simulink model "PrimaryController"  (R2023a)
settings: Solver=VariableStepAuto  StartTime=0.0  StopTime=inf  RelTol=1e-3
model workspace (MAT data in the model file):
  MyTestVariable = Simulink.Parameter
  MyTestVariable.Value = 5
  MyTestVariable.DataType = 'auto'
  MyTestVariable.Min = 1
  MyTestVariable.Max = 10
  MyTestVariable.Complexity = 'real'
  MyTestVariable.Dimensions = [1 1]
libraries: arduinolib x20, simulink x2
settings Model: Creator=Josh Lendi  LastModifiedBy=alanl
settings DebuggingCC: UnconnectedInputMsg=warning  UnconnectedOutputMsg=warning  UnconnectedLineMsg=warning
settings ModelReferenceCC: EnableRefExpFcnMdlSchedulingChecks=on
settings RTWCC: DLArmComputeVersion=19.05

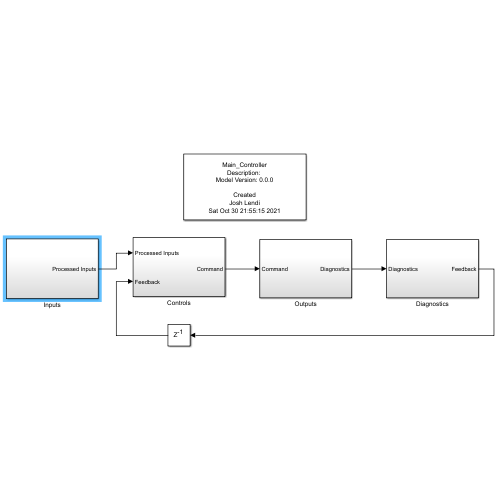
[thumbnail: Simulink's stored preview of the top-level diagram]
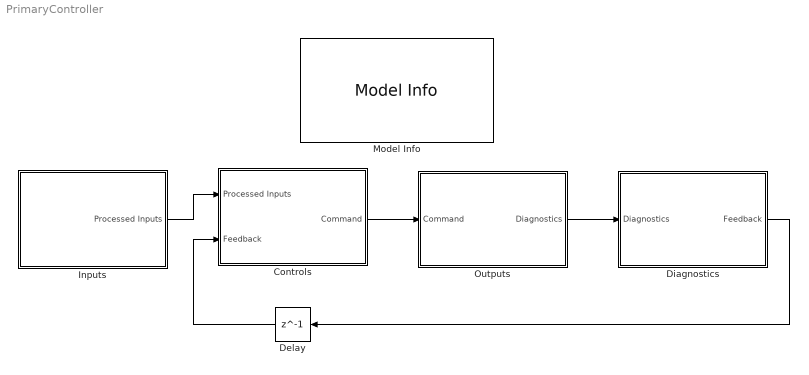
== system PrimaryController ==
  Controls : Subsystem
  Delay : Delay  DelayLength=1  InitialCondition=0
  Diagnostics : Subsystem
  Inputs : Subsystem
  Model Info : simulink/Model-Wide Utilities/Model Info  Frame=on  DisplayStringWithTags=|  HorizontalTextAlignment=Center  LeftAlignmentValue=0.5
      | %<ModelName>
      | Description: %<Description>
      | Model Version: %<ModelVersion>
      | 
      | Created
      | %<Creator>
      | %<Created>
  Outputs : Subsystem
  wires:
  Controls/1(Command) -> Outputs/1(Command)
  Outputs/1(Diagnostics) -> Diagnostics/1(Diagnostics)
  Inputs/1(Processed Inputs) -> Controls/1(Processed Inputs)
  Delay/1 -> Controls/2(Feedback)
  Diagnostics/1(Feedback) -> Delay/1

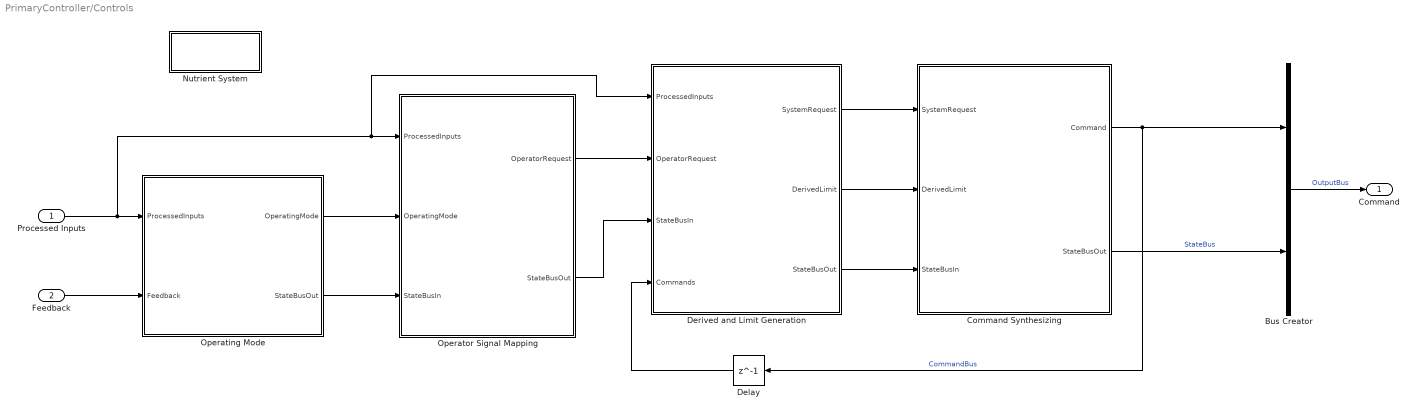
== system PrimaryController/Controls ==
  Processed Inputs : Inport
  Feedback : Inport  Port=2
  Bus Creator : BusCreator  Inputs=2
  Command Synthesizing : Subsystem
  Delay : Delay  DelayLength=1
  Derived and Limit Generation : Subsystem
  Nutrient System : Subsystem
  Operating Mode : Subsystem
  Operator Signal Mapping : Subsystem
  Command : Outport
  wires:
  Processed Inputs/1 -> Derived and Limit Generation/1(ProcessedInputs), Operator Signal Mapping/1(ProcessedInputs), Operating Mode/1(ProcessedInputs)
  Feedback/1 -> Operating Mode/2(Feedback)
  Operating Mode/1(OperatingMode) -> Operator Signal Mapping/2(OperatingMode)
  Operating Mode/2(StateBusOut) -> Operator Signal Mapping/3(StateBusIn)
  Operator Signal Mapping/1(OperatorRequest) -> Derived and Limit Generation/2(OperatorRequest)
  Operator Signal Mapping/2(StateBusOut) -> Derived and Limit Generation/3(StateBusIn)
  Derived and Limit Generation/1(SystemRequest) -> Command Synthesizing/1(SystemRequest)
  Derived and Limit Generation/2(DerivedLimit) -> Command Synthesizing/2(DerivedLimit)
  Derived and Limit Generation/3(StateBusOut) -> Command Synthesizing/3(StateBusIn)
  Command Synthesizing/2(StateBusOut) -> Bus Creator/2  "StateBus"
  Command Synthesizing/1(Command) -> Delay/1, Bus Creator/1  "CommandBus"
  Bus Creator/1 -> Command/1  "OutputBus"
  Delay/1 -> Derived and Limit Generation/4(Commands)

== system PrimaryController/Diagnostics ==
  Diagnostics : Inport
  Feedback : Outport
  wires:
  Diagnostics/1 -> Feedback/1

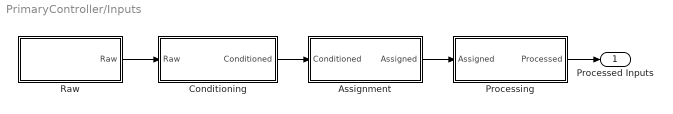
== system PrimaryController/Inputs ==
  Assignment : Subsystem
  Conditioning : Subsystem
  Processing : Subsystem
  Raw : Subsystem
  Processed Inputs : Outport
  wires:
  Raw/1(Raw) -> Conditioning/1(Raw)
  Assignment/1(Assigned) -> Processing/1(Assigned)
  Conditioning/1(Conditioned) -> Assignment/1(Conditioned)
  Processing/1(Processed) -> Processed Inputs/1

== system PrimaryController/Outputs ==
  Command : Inport
  Processing : Subsystem
  Send : Subsystem
  Diagnostics : Outport
  wires:
  Command/1 -> Processing/1(Command)
  Send/1(Diagnostic) -> Diagnostics/1
  Processing/1(Processed) -> Send/1(Processed)

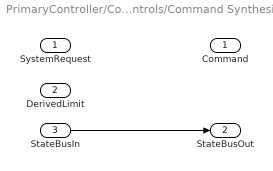
== system PrimaryController/Controls/Command Synthesizing ==
  SystemRequest : Inport
  DerivedLimit : Inport  Port=2
  StateBusIn : Inport  Port=3
  Command : Outport
  StateBusOut : Outport  Port=2
  wires:
  StateBusIn/1 -> StateBusOut/1

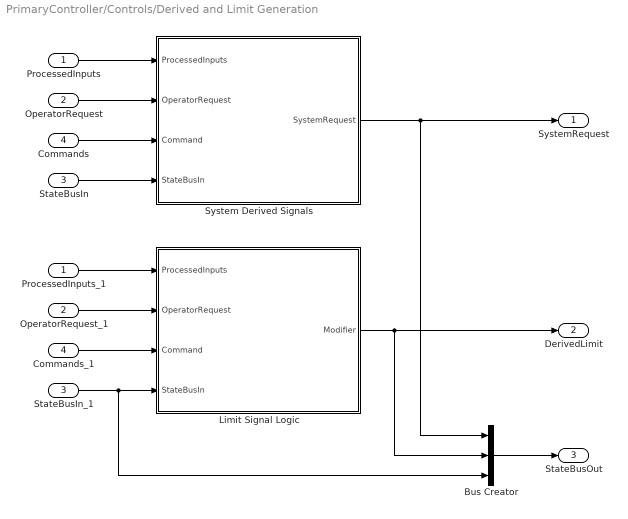
== system PrimaryController/Controls/Derived and Limit Generation ==
  ProcessedInputs : Inport
  OperatorRequest : Inport  Port=2
  StateBusIn : Inport  Port=3
  Commands : Inport  Port=4
  Bus Creator : BusCreator  Inputs=3
  Commands_1 : InportShadow  Port=4
  Limit Signal Logic : Subsystem
  OperatorRequest_1 : InportShadow  Port=2
  ProcessedInputs_1 : InportShadow
  StateBusIn_1 : InportShadow  Port=3
  System Derived Signals : Subsystem
  SystemRequest : Outport
  DerivedLimit : Outport  Port=2
  StateBusOut : Outport  Port=3
  wires:
  ProcessedInputs/1 -> System Derived Signals/1(ProcessedInputs)
  OperatorRequest/1 -> System Derived Signals/2(OperatorRequest)
  Commands/1 -> System Derived Signals/3(Command)
  StateBusIn/1 -> System Derived Signals/4(StateBusIn)
  ProcessedInputs_1/1 -> Limit Signal Logic/1(ProcessedInputs)
  OperatorRequest_1/1 -> Limit Signal Logic/2(OperatorRequest)
  Commands_1/1 -> Limit Signal Logic/3(Command)
  StateBusIn_1/1 -> Limit Signal Logic/4(StateBusIn), Bus Creator/3
  Limit Signal Logic/1(Modifier) -> DerivedLimit/1, Bus Creator/2
  System Derived Signals/1(SystemRequest) -> SystemRequest/1, Bus Creator/1
  Bus Creator/1 -> StateBusOut/1

== system PrimaryController/Controls/Nutrient System ==
  TDS Measurement : Subsystem
  pH Increase Pump : Stateflow chart  TreatAsAtomicUnit=on
  pH Measurement : Subsystem

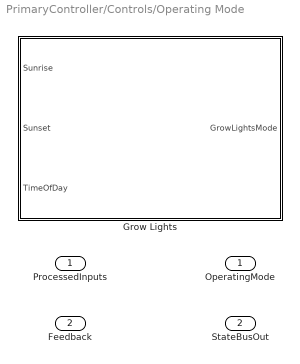
== system PrimaryController/Controls/Operating Mode ==
  ProcessedInputs : Inport
  Feedback : Inport  Port=2
  Grow Lights : Stateflow chart  TreatAsAtomicUnit=on
  OperatingMode : Outport
  StateBusOut : Outport  Port=2

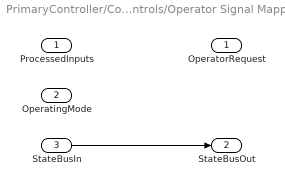
== system PrimaryController/Controls/Operator Signal Mapping ==
  ProcessedInputs : Inport
  OperatingMode : Inport  Port=2
  StateBusIn : Inport  Port=3
  OperatorRequest : Outport
  StateBusOut : Outport  Port=2
  wires:
  StateBusIn/1 -> StateBusOut/1

== system PrimaryController/Inputs/Assignment ==
  Conditioned : Inport
  Assigned : Outport
  wires:
  Conditioned/1 -> Assigned/1

== system PrimaryController/Inputs/Conditioning ==
  Raw : Inport
  Conditioned : Outport
  wires:
  Raw/1 -> Conditioned/1

== system PrimaryController/Inputs/Processing ==
  Assigned : Inport
  Processed : Outport
  wires:
  Assigned/1 -> Processed/1

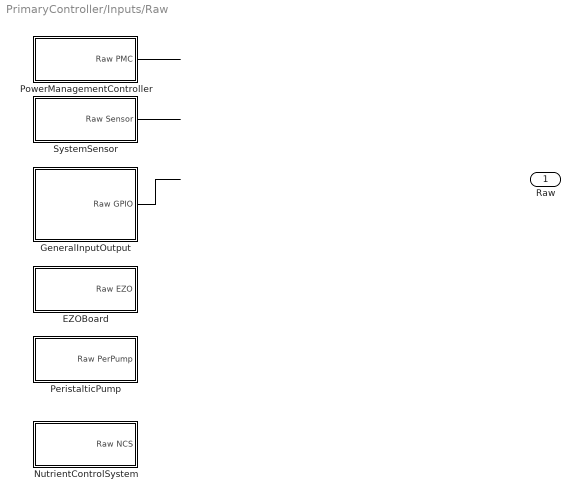
== system PrimaryController/Inputs/Raw ==
  EZOBoard : Subsystem
  GeneralInputOutput : Subsystem
  NutrientControlSystem : Subsystem
  PeristalticPump : Subsystem
  PowerManagementController : Subsystem
  SystemSensor : Subsystem
  Raw : Outport
  wires:
  GeneralInputOutput/1(Raw GPIO) -> ?
  PowerManagementController/1(Raw PMC) -> ?
  SystemSensor/1(Raw Sensor) -> ?

== system PrimaryController/Outputs/Processing ==
  Command : Inport
  Processed : Outport
  wires:
  Command/1 -> Processed/1

== system PrimaryController/Outputs/Send ==
  Processed : Inport
  Diagnostic : Outport
  wires:
  Processed/1 -> Diagnostic/1

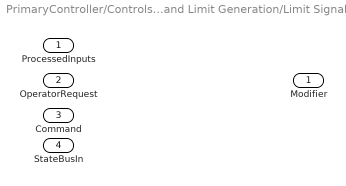
== system PrimaryController/Controls/Derived and Limit Generation/Limit Signal Logic ==
  ProcessedInputs : Inport
  OperatorRequest : Inport  Port=2
  Command : Inport  Port=3
  StateBusIn : Inport  Port=4
  Modifier : Outport

== system PrimaryController/Controls/Derived and Limit Generation/System Derived Signals ==
  ProcessedInputs : Inport
  OperatorRequest : Inport  Port=2
  Command : Inport  Port=3
  StateBusIn : Inport  Port=4
  SystemRequest : Outport

== system PrimaryController/Controls/Nutrient System/TDS Measurement ==
  In1 : Inport
  Out1 : Outport
  wires:
  In1/1 -> Out1/1

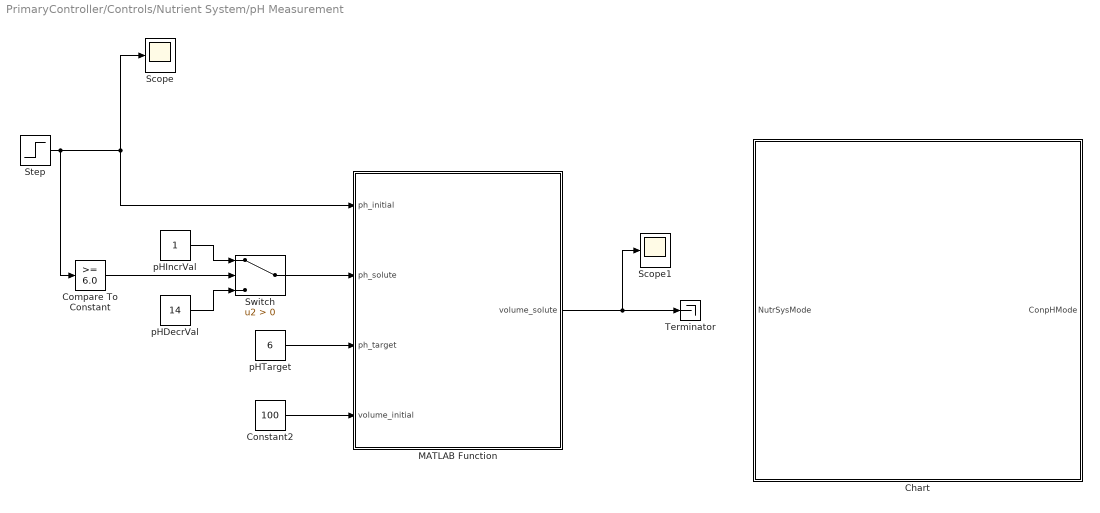
== system PrimaryController/Controls/Nutrient System/pH Measurement ==
  Chart : Stateflow chart  TreatAsAtomicUnit=on
  Compare To Constant : simulink/Logic and Bit Operations/Compare To Constant  relop=>=  const=6.0  OutDataTypeStr=boolean
  Constant2 : Constant  Value=100
  MATLAB Function : MATLAB Function  TreatAsAtomicUnit=on
  Scope : Scope
  Scope1 : Scope
  Step : Step  Before=6  After=7  SampleTime=0
  Switch : Switch  Criteria=u2 > Threshold  SaturateOnIntegerOverflow=off  InputSameDT=off
  Terminator : Terminator
  pHDecrVal : Constant  Value=14
  pHIncrVal : Constant
  pHTarget : Constant  Value=6
  wires:
  pHIncrVal/1 -> Switch/1
  pHTarget/1 -> MATLAB Function/3(ph_target)
  Step/1 -> Scope/1, MATLAB Function/1(ph_initial), Compare To Constant/1
  MATLAB Function/1(volume_solute) -> Scope1/1, Terminator/1
  Constant2/1 -> MATLAB Function/4(volume_initial)
  pHDecrVal/1 -> Switch/3
  Compare To Constant/1 -> Switch/2
  Switch/1 -> MATLAB Function/2(ph_solute)

== system PrimaryController/Inputs/Raw/EZOBoard ==
  Raw EZO : Outport

== system PrimaryController/Inputs/Raw/GeneralInputOutput ==
  Bus Creator : BusCreator  Inputs=15
  Raw GPIO : Outport
  wires:
  Bus Creator/1 -> Raw GPIO/1

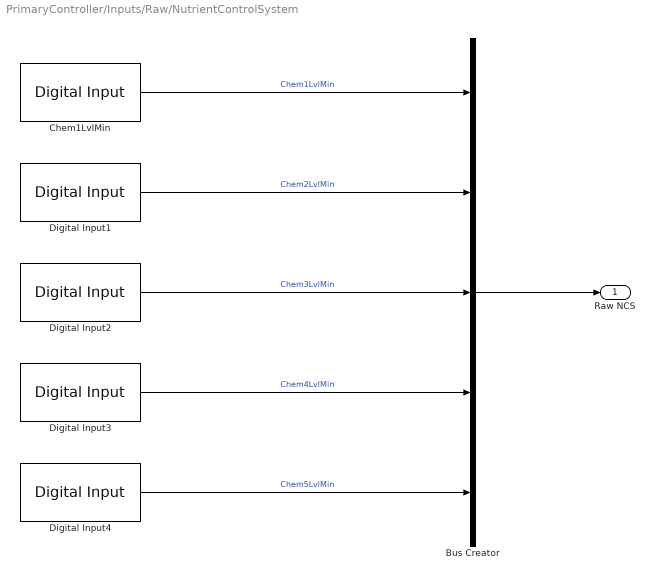
== system PrimaryController/Inputs/Raw/NutrientControlSystem ==
  Bus Creator : BusCreator  Inputs=5
  Chem1LvlMin : arduinolib/Digital Input  pinNumber=8  mode=Default  Direction=input  SampleTime=0.1  blockPlatform=arduino
  Digital Input{1..4} (4 alike) : arduinolib/Digital Input  pinNumber=8  mode=Default  Direction=input  SampleTime=0.1  blockPlatform=arduino
  Raw NCS : Outport
  wires:
  Digital Input4/1 -> Bus Creator/5  "Chem5LvlMin"
  Digital Input3/1 -> Bus Creator/4  "Chem4LvlMin"
  Digital Input2/1 -> Bus Creator/3  "Chem3LvlMin"
  Digital Input1/1 -> Bus Creator/2  "Chem2LvlMin"
  Chem1LvlMin/1 -> Bus Creator/1  "Chem1LvlMin"
  Bus Creator/1 -> Raw NCS/1

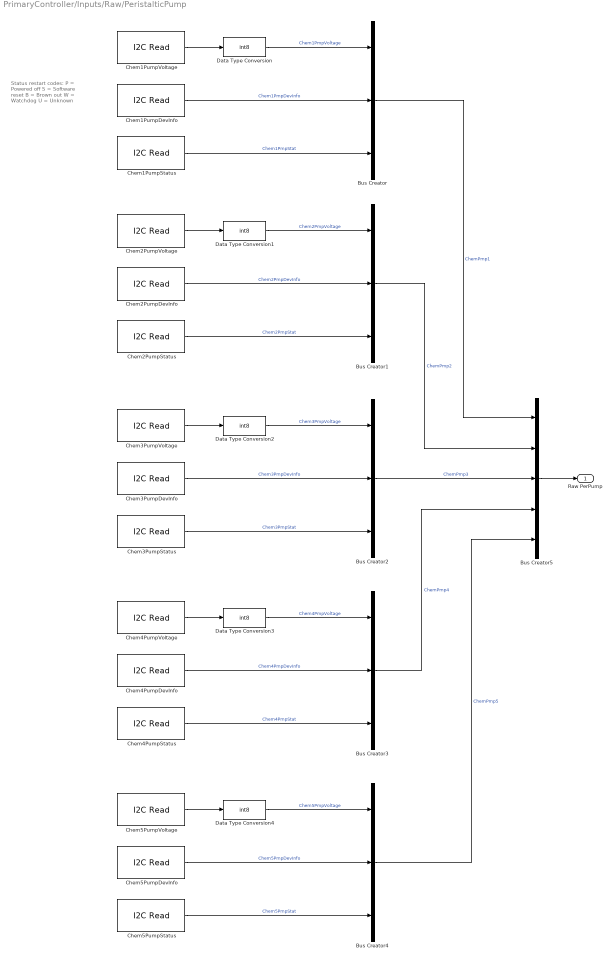
== system PrimaryController/Inputs/Raw/PeristalticPump ==
  note: Status restart codes:
      | P = Powered off
      | S = Software reset
      | B = Brown out
      | W = Watchdog
      | U = Unknown
  Bus Creator{,1..4} (5 alike) : BusCreator  Inputs=3
  Bus Creator5 : BusCreator  Inputs=5
  Chem1PumpDevInfo : arduinolib/I2C Read  I2CModule=0  Mode=Master  SlaveAddress=10  SlaveByteOrder=BigEndian  Direction=Receiver  RegisterAddressMode=on  RegisterAddress=0  SlaveDataType=uint8  DataLength=1  NoAck=off  RepeatedStart=off  OutputStatus=off  blockPlatform=ARDUINO  SampleTime=0.1
  Chem1PumpStatus : arduinolib/I2C Read  I2CModule=0  Mode=Master  SlaveAddress=10  SlaveByteOrder=BigEndian  Direction=Receiver  RegisterAddressMode=on  RegisterAddress=0  SlaveDataType=uint8  DataLength=1  NoAck=off  RepeatedStart=off  OutputStatus=off  blockPlatform=ARDUINO  SampleTime=0.1
  Chem1PumpVoltage : arduinolib/I2C Read  I2CModule=0  Mode=Master  SlaveAddress=10  SlaveByteOrder=BigEndian  Direction=Receiver  RegisterAddressMode=on  RegisterAddress=0  SlaveDataType=uint8  DataLength=1  NoAck=off  RepeatedStart=off  OutputStatus=off  blockPlatform=ARDUINO  SampleTime=0.1
  Chem2PumpDevInfo : arduinolib/I2C Read  I2CModule=0  Mode=Master  SlaveAddress=10  SlaveByteOrder=BigEndian  Direction=Receiver  RegisterAddressMode=on  RegisterAddress=0  SlaveDataType=uint8  DataLength=1  NoAck=off  RepeatedStart=off  OutputStatus=off  blockPlatform=ARDUINO  SampleTime=0.1
  Chem2PumpStatus : arduinolib/I2C Read  I2CModule=0  Mode=Master  SlaveAddress=10  SlaveByteOrder=BigEndian  Direction=Receiver  RegisterAddressMode=on  RegisterAddress=0  SlaveDataType=uint8  DataLength=1  NoAck=off  RepeatedStart=off  OutputStatus=off  blockPlatform=ARDUINO  SampleTime=0.1
  Chem2PumpVoltage : arduinolib/I2C Read  I2CModule=0  Mode=Master  SlaveAddress=10  SlaveByteOrder=BigEndian  Direction=Receiver  RegisterAddressMode=on  RegisterAddress=0  SlaveDataType=uint8  DataLength=1  NoAck=off  RepeatedStart=off  OutputStatus=off  blockPlatform=ARDUINO  SampleTime=0.1
  Chem3PumpDevInfo : arduinolib/I2C Read  I2CModule=0  Mode=Master  SlaveAddress=10  SlaveByteOrder=BigEndian  Direction=Receiver  RegisterAddressMode=on  RegisterAddress=0  SlaveDataType=uint8  DataLength=1  NoAck=off  RepeatedStart=off  OutputStatus=off  blockPlatform=ARDUINO  SampleTime=0.1
  Chem3PumpStatus : arduinolib/I2C Read  I2CModule=0  Mode=Master  SlaveAddress=10  SlaveByteOrder=BigEndian  Direction=Receiver  RegisterAddressMode=on  RegisterAddress=0  SlaveDataType=uint8  DataLength=1  NoAck=off  RepeatedStart=off  OutputStatus=off  blockPlatform=ARDUINO  SampleTime=0.1
  Chem3PumpVoltage : arduinolib/I2C Read  I2CModule=0  Mode=Master  SlaveAddress=10  SlaveByteOrder=BigEndian  Direction=Receiver  RegisterAddressMode=on  RegisterAddress=0  SlaveDataType=uint8  DataLength=1  NoAck=off  RepeatedStart=off  OutputStatus=off  blockPlatform=ARDUINO  SampleTime=0.1
  Chem4PumpDevInfo : arduinolib/I2C Read  I2CModule=0  Mode=Master  SlaveAddress=10  SlaveByteOrder=BigEndian  Direction=Receiver  RegisterAddressMode=on  RegisterAddress=0  SlaveDataType=uint8  DataLength=1  NoAck=off  RepeatedStart=off  OutputStatus=off  blockPlatform=ARDUINO  SampleTime=0.1
  Chem4PumpStatus : arduinolib/I2C Read  I2CModule=0  Mode=Master  SlaveAddress=10  SlaveByteOrder=BigEndian  Direction=Receiver  RegisterAddressMode=on  RegisterAddress=0  SlaveDataType=uint8  DataLength=1  NoAck=off  RepeatedStart=off  OutputStatus=off  blockPlatform=ARDUINO  SampleTime=0.1
  Chem4PumpVoltage : arduinolib/I2C Read  I2CModule=0  Mode=Master  SlaveAddress=10  SlaveByteOrder=BigEndian  Direction=Receiver  RegisterAddressMode=on  RegisterAddress=0  SlaveDataType=uint8  DataLength=1  NoAck=off  RepeatedStart=off  OutputStatus=off  blockPlatform=ARDUINO  SampleTime=0.1
  Chem5PumpDevInfo : arduinolib/I2C Read  I2CModule=0  Mode=Master  SlaveAddress=10  SlaveByteOrder=BigEndian  Direction=Receiver  RegisterAddressMode=on  RegisterAddress=0  SlaveDataType=uint8  DataLength=1  NoAck=off  RepeatedStart=off  OutputStatus=off  blockPlatform=ARDUINO  SampleTime=0.1
  Chem5PumpStatus : arduinolib/I2C Read  I2CModule=0  Mode=Master  SlaveAddress=10  SlaveByteOrder=BigEndian  Direction=Receiver  RegisterAddressMode=on  RegisterAddress=0  SlaveDataType=uint8  DataLength=1  NoAck=off  RepeatedStart=off  OutputStatus=off  blockPlatform=ARDUINO  SampleTime=0.1
  Chem5PumpVoltage : arduinolib/I2C Read  I2CModule=0  Mode=Master  SlaveAddress=10  SlaveByteOrder=BigEndian  Direction=Receiver  RegisterAddressMode=on  RegisterAddress=0  SlaveDataType=uint8  DataLength=1  NoAck=off  RepeatedStart=off  OutputStatus=off  blockPlatform=ARDUINO  SampleTime=0.1
  Data Type Conversion{,1..4} (5 alike) : DataTypeConversion  OutDataTypeStr=int8  SaturateOnIntegerOverflow=off  RndMeth=Floor  LockScale=on
  Raw PerPump : Outport
  wires:
  Chem1PumpVoltage/1 -> Data Type Conversion/1
  Bus Creator5/1 -> Raw PerPump/1
  Data Type Conversion/1 -> Bus Creator/1  "Chem1PmpVoltage"
  Chem1PumpDevInfo/1 -> Bus Creator/2  "Chem1PmpDevInfo"
  Chem1PumpStatus/1 -> Bus Creator/3  "Chem1PmpStat"
  Data Type Conversion1/1 -> Bus Creator1/1  "Chem2PmpVoltage"
  Chem2PumpDevInfo/1 -> Bus Creator1/2  "Chem2PmpDevInfo"
  Chem2PumpStatus/1 -> Bus Creator1/3  "Chem2PmpStat"
  Chem2PumpVoltage/1 -> Data Type Conversion1/1
  Data Type Conversion2/1 -> Bus Creator2/1  "Chem3PmpVoltage"
  Chem3PumpDevInfo/1 -> Bus Creator2/2  "Chem3PmpDevInfo"
  Chem3PumpStatus/1 -> Bus Creator2/3  "Chem3PmpStat"
  Chem3PumpVoltage/1 -> Data Type Conversion2/1
  Chem4PumpStatus/1 -> Bus Creator3/3  "Chem4PmpStat"
  Chem4PumpDevInfo/1 -> Bus Creator3/2  "Chem4PmpDevInfo"
  Data Type Conversion3/1 -> Bus Creator3/1  "Chem4PmpVoltage"
  Chem4PumpVoltage/1 -> Data Type Conversion3/1
  Chem5PumpStatus/1 -> Bus Creator4/3  "Chem5PmpStat"
  Data Type Conversion4/1 -> Bus Creator4/1  "Chem5PmpVoltage"
  Chem5PumpVoltage/1 -> Data Type Conversion4/1
  Chem5PumpDevInfo/1 -> Bus Creator4/2  "Chem5PmpDevInfo"
  Bus Creator2/1 -> Bus Creator5/3  "ChemPmp3"
  Bus Creator3/1 -> Bus Creator5/4  "ChemPmp4"
  Bus Creator4/1 -> Bus Creator5/5  "ChemPmp5"
  Bus Creator1/1 -> Bus Creator5/2  "ChemPmp2"
  Bus Creator/1 -> Bus Creator5/1  "ChemPmp1"

== system PrimaryController/Inputs/Raw/PowerManagementController ==
  Raw PMC : Outport

== system PrimaryController/Inputs/Raw/SystemSensor ==
  Bus Creator : BusCreator  Inputs=5
  Raw Sensor : Outport
  wires:
  Bus Creator/1 -> Raw Sensor/1

== stateflow chart PrimaryController/Controls/Nutrient System/pH Increase Pump ==
  state Device Information
  state Calibration
  state Report
  state Dispense
    state Continuous
    state Volume
    state Dose
    state ConstantFlow
    (default) -> Continuous
  state Pause
  state Stop
  state Sleep
  (default) -> Device Information

== matlab function PrimaryController/Controls/Nutrient System/pH Measurement/MATLAB Function ==
  data: ph_initial input; volume_solute output; ph_solute input; ph_target input; volume_initial input
function volume_solute = pHNeutralization(ph_initial, ph_solute, ph_target, volume_initial)
    %Molarity
    M_initial = 10^(-ph_initial); %Initial molarity of solution
    M_solute = 10^(-ph_solute); %Fixed molarity of solute
    M_target = 10^(-ph_target); %Final or target molarity of solution
    
    
volume_solute = (M_target*volume_initial - M_initial*volume_initial)/(M_solute-M_target);

== stateflow chart PrimaryController/Controls/Nutrient System/pH Measurement/Chart ==
  state Measurement
    ConpHMode=2;
  state Sleep
    ConpHMode=1;
  state Calibration
    ConpHMode=3;
  (default) -> Measurement
  Measurement -> Sleep [order 1] : [ConpHMode==1]
  Sleep -> Measurement : [ConpHMode==2]
  Measurement -> Calibration [order 2] : [ConpHMode==3]
  data: ConpHMode output; NutrSysMode input

== stateflow chart PrimaryController/Controls/Operating Mode/Grow Lights ==
  state Morning
    GrowLightsMode=1;
  state Midday
    GrowLightsMode=2;
  state Afternoon
    GrowLightsMode=3;
  state Night
    GrowLightsMode=4;
  (default) -> Morning
  Night -> Morning : [TimeOfDay==Sunrise]
  Morning -> Midday : [TimeOfDay>=11]
  Midday -> Afternoon : [TimeOfDay>=13]
  Afternoon -> Night : [TimeOfDay==Sunset]
  data: GrowLightsMode output; Sunrise input; Sunset input; TimeOfDay input
